simulink model "C28069_LLC_ePWM_V8_230307_PhaeShiftWorking"  (R2022b)
settings: Solver=FixedStepAuto  StartTime=0.0  StopTime=10  RelTol=1e-3  EnableMultiTasking=on
model workspace (MAT data in the model file):
  Comp_DAC = 512
undefined symbols (not defined in the file or in its folder): Down, GPTRIP1SEL, GPTRIP2SEL, PWM_Control, PWM_Gen, PWM_Gen1, SCI_A_Transmit, SCI_A_Transmit_Current_Suffix, SCI_A_Transmit_Duty_Suffix, SCI_A_Transmit_Freq_Suffix, SCI_A_Transmit_OVPFlag_Suffix, SCI_A_Transmit_PFC_Suffix, SCI_A_Transmit_SS_Suffix, SCI_A_Transmit_TBPHS_Suffix, SCI_A_Transmit_VADC_Suffix, SCI_A_Transmit_VAvg_Suffix, SCI_A_Transmit_VBAT_Suffix, SCI_A_Transmit_VBATRef_Suffix, SCI_A_Transmit_Vo_Suffix, TZ1, TZ2, u1, Up
libraries: c2802xlib x92, c280xlib x39, simulink x36, c2000lib x1
(part 2 of 18)

== system C28069_LLC_ePWM_V8_230307_PhaeShiftWorking/Simulink Function1 ==
  note: Added Trigger
  note: Fixing deadtime to 250ns
  note: Control CMPA/B to Zero
      | When the input is <1KHz
      | (To switch off ePWM)
  note: Frequency Input Selection
  note: Original
  PWM_Gen : TriggerPort  TriggerType=function-call  IsSimulinkFunction=on  FunctionName=PWM_Gen  FunctionVisibility=scoped  VariantControl=(inherit)
  CMPA : Display
  CMPA1 : Display
  CMPB : Display
  CMPB1 : Display
  Constant : Constant  Value=100
  Constant1 : Constant
  Constant2 : Constant
  Constant4 : Constant
  Dead time (%) : Display
  Dead time (sec) : Constant  Value=250E-9
  Divide : Product  Inputs=*/
  Gain : Gain  Gain=100
  Gain1 : Gain  Gain=1000
  Product{1..4} (4 alike) : Product
  Subsystem : Subsystem
  Subtract : Sum  Inputs=+-
  Switch : Switch  Criteria=u2 > Threshold  Threshold=1  SaturateOnIntegerOverflow=off  InputSameDT=off
  Switch1 : Switch  Criteria=u2 > Threshold  SaturateOnIntegerOverflow=off  InputSameDT=off
  TBPRD : Display
  ePWM1 : c2802xlib/ePWM  PwmType=C2000  useModule=ePWM6  ePWMxLINKTBPRD=Not Linked  periodUnits=Clock cycles  timerSource=Input port  timerPeriod_clk=294  timerPeriod_sec=0.0001  tbshadow=Counter equals to zero  countingMode=Up-Down  phaseActiveEnable=Disable  phaseDirection=Count down after sync  phaseActive=0  synchronizationEnable=off  dcaevt1Sync=off  dcbevt1Sync=off  synchronizationOption=Disable  dcbevt1SyncOut=off  dcaevt1SyncOut=off  cmpdSyncOut=off  cmpcSyncOut=off  cmpbSyncOut=off  zeroSyncOut=off  swfSyncOut=off  perSynchronizationOption=Counter equals to period (CTR=PRD)  clockPrescale=1  HSclockPrescale=1  enswap=off  ePWMxAStatus=on  ePWMxAactionLogic1=Do nothing  ePWMxAactionLogic2=Do nothing  ePWMxAactionLogic3=Set  ePWMxAactionLogic4=Do nothing  ePWMxAactionLogic5=Clear  ePWMxAactionLogic6=Do nothing  ePWMxACSFenable=off  ePWMxACSFvalue=Forcing disable  ePWMxASFreload=Zero  ePWMxBStatus=on  ePWMxBactionLogic1=Do nothing  ePWMxBactionLogic2=Do nothing  ePWMxBactionLogic3=Do nothing  ePWMxBactionLogic4=Clear  ePWMxBactionLogic5=Do nothing  ePWMxBactionLogic6=Set  ePWMxBCSFenable=off  ePWMxBCSFvalue=Forcing disable  ePWMxBSFreload=Zero  ePWNxBOutWay=off  ePWMxLINKCMPA=Not Linked  CMPAUnits=Clock cycles  CMPASource=Input port  CMPAValue_per=50  CMPAValue_clk=12  enCMPAshadow=Counter equals to zero (CTR=Zero)  ePWMxLINKCMPB=Not Linked  CMPBUnits=Clock cycles  CMPBSource=Input port  CMPBValue_per=50  CMPBValue_clk=283  enCMPBshadow=Counter equals to zero (CTR=Zero)  ePWMxLINKCMPC=Not Linked  CMPCUnits=Clock cycles  CMPCSource=Specify via dialog  CMPCValue_per=50  CMPCValue_clk=32000  enCMPCshadow=Counter equals to zero (CTR=Zero)  ePWMxLINKCMPD=Not Linked  CMPDUnits=Clock cycles  CMPDSource=Specify via dialog  CMPDValue_per=50  CMPDValue_clk=32000  enCMPDshadow=Counter equals to zero (CTR=Zero)  enableDBePWMxA=off  enableDBePWMxB=off  enhalfcycle=off  DBpolarity=Active high complementary (AHC)  DBedgeDelay=Positive  DBSource_ePWMxA=ePWMxA  DBSource_ePWMxB=ePWMxA  DBPeriodUnits=Clock cycles  DBperiodSource=Input port  REDperiod=10  FEDperiod=10  REDperiod_sec=0  FEDperiod_sec=0  LoadModeDBRED=Immediate without using shadow  LoadModeDBFED=Immediate without using shadow  adcstartModuleA=off  adcrequestEventA=First event  adcstartEventA=Counter equals to zero (CTR=Zero)  adcstartEventA_type2=Digital Compare Module A Event 1 start of conversion (DCAEVT1.soc)  adcstartModuleB=off  adcrequestEventB=First event  adcstartEventB=Counter equals to zero (CTR=Zero)  adcstartEventB_type2=Counter equals to zero (CTR=Zero)  intEn=off  intPrd=First event  intSel=Counter equals to zero (CTR=Zero)  intSel_type2=Counter equals to zero (CTR=Zero)  hrpe=off  enHRPWM=off  HRPWM_LoadMode=Counter equals to period (CTR=PRD)  HRPWM_CTLMode=Duty or Period control mode  HRPWM_EDGMode=Both edge  hrpeb=off  enHRPWMB=off  HRPWM_LoadModeB=Counter equals to zero (CTR=ZERO)  HRPWM_CTLModeB=Duty or Period control mode  HRPWM_EDGModeB=Both edge  enHRDBRED=off  enHRDBFED=off  enSFO=on  enautoconv=on  chopperEnable=off  chopperFrequency=1  chopperFirstwidth=1  chopperDuty=12.5%  tripZonesource=Specify via dialog  tzselOSHT1=off  tzselOSHT2=off  tzselOSHT3=off  tzselOSHDCAEV1=off  tzselOSHDCBEV1=off  tzselCBC1=off  tzselCBC2=off  tzselCBC3=off  tzselCBCDCAEV2=off  tzselCBCDCBEV2=off  tzselOSHT4=off  tzselOSHT5=off  tzselOSHT6=off  tzselCBC4=off  tzselCBC5=off  tzselCBC6=off  enTzOstIntr=off  enTzCbcIntr=off  enTzDCAEVT1Intr=off  enTzDCAEVT2Intr=off  enTzDCBEVT1Intr=off  enTzDCBEVT2Intr=off  ePWMxAforced=No action  ePWMxBforced=No action  DCAEVT1forced=Low  DCBEVT1forced=Low  DCAEVT2forced=No action  DCBEVT2forced=No action  dcah=COMP1OUT input  dcal=Trip Zone 1 input (TZ1)  dcbh=COMP1OUT input  dcbl=Trip Zone 1 input (TZ1)  dcah_type2=GPTRIP1SEL/(TZ1)  dcal_type2=GPTRIP2SEL/(TZ2)  dcbh_type2=GPTRIP1SEL/(TZ1)  dcbl_type2=GPTRIP2SEL/(TZ2)  gendcaevt1=DCAH=high and DCAL=don't care  gendcaevt2=Event disabled  gendcbevt1=DCBH=high and DCBL=don't care  gendcbevt2=Event disabled  dcaevt1src=DCAEVT1 with sync  dcaevt2src=DCAEVT2 with sync  dcbevt1src=DCBEVT1 with sync  dcbevt2src=DCBEVT2 with sync  pulsesel=Counter equals to zero (CTR=Zero)  blankinv=off  blankoffset=0  blankwidth=0  evsrcsel=Filtered version of DCAEVT1 (DCAEVT1FILT)  encape=off
      settings: LibrarySourceBlock=c2806xlib/ePWM
  ePWM4 : c2802xlib/ePWM  PwmType=C2000  useModule=ePWM5  ePWMxLINKTBPRD=Not Linked  periodUnits=Clock cycles  timerSource=Input port  timerPeriod_clk=294  timerPeriod_sec=0.0001  tbshadow=Counter equals to zero  countingMode=Up-Down  phaseActiveEnable=Disable  phaseDirection=Count down after sync  phaseActive=0  synchronizationEnable=off  dcaevt1Sync=off  dcbevt1Sync=off  synchronizationOption=Disable  dcbevt1SyncOut=off  dcaevt1SyncOut=off  cmpdSyncOut=off  cmpcSyncOut=off  cmpbSyncOut=off  zeroSyncOut=off  swfSyncOut=off  perSynchronizationOption=Counter equals to period (CTR=PRD)  clockPrescale=1  HSclockPrescale=1  enswap=off  ePWMxAStatus=on  ePWMxAactionLogic1=Do nothing  ePWMxAactionLogic2=Do nothing  ePWMxAactionLogic3=Set  ePWMxAactionLogic4=Do nothing  ePWMxAactionLogic5=Clear  ePWMxAactionLogic6=Do nothing  ePWMxACSFenable=off  ePWMxACSFvalue=Forcing disable  ePWMxASFreload=Zero  ePWMxBStatus=on  ePWMxBactionLogic1=Do nothing  ePWMxBactionLogic2=Do nothing  ePWMxBactionLogic3=Do nothing  ePWMxBactionLogic4=Clear  ePWMxBactionLogic5=Do nothing  ePWMxBactionLogic6=Set  ePWMxBCSFenable=off  ePWMxBCSFvalue=Forcing disable  ePWMxBSFreload=Zero  ePWNxBOutWay=off  ePWMxLINKCMPA=Not Linked  CMPAUnits=Clock cycles  CMPASource=Input port  CMPAValue_per=50  CMPAValue_clk=12  enCMPAshadow=Counter equals to zero (CTR=Zero)  ePWMxLINKCMPB=Not Linked  CMPBUnits=Clock cycles  CMPBSource=Input port  CMPBValue_per=50  CMPBValue_clk=283  enCMPBshadow=Counter equals to zero (CTR=Zero)  ePWMxLINKCMPC=Not Linked  CMPCUnits=Clock cycles  CMPCSource=Specify via dialog  CMPCValue_per=50  CMPCValue_clk=32000  enCMPCshadow=Counter equals to zero (CTR=Zero)  ePWMxLINKCMPD=Not Linked  CMPDUnits=Clock cycles  CMPDSource=Specify via dialog  CMPDValue_per=50  CMPDValue_clk=32000  enCMPDshadow=Counter equals to zero (CTR=Zero)  enableDBePWMxA=off  enableDBePWMxB=off  enhalfcycle=off  DBpolarity=Active high complementary (AHC)  DBedgeDelay=Positive  DBSource_ePWMxA=ePWMxA  DBSource_ePWMxB=ePWMxA  DBPeriodUnits=Clock cycles  DBperiodSource=Input port  REDperiod=10  FEDperiod=10  REDperiod_sec=0  FEDperiod_sec=0  LoadModeDBRED=Immediate without using shadow  LoadModeDBFED=Immediate without using shadow  adcstartModuleA=on  adcrequestEventA=First event  adcstartEventA=Counter equals to zero (CTR=Zero)  adcstartEventA_type2=Digital Compare Module A Event 1 start of conversion (DCAEVT1.soc)  adcstartModuleB=off  adcrequestEventB=First event  adcstartEventB=Counter equals to zero (CTR=Zero)  adcstartEventB_type2=Counter equals to zero (CTR=Zero)  intEn=on  intPrd=First event  intSel=Counter equals to zero (CTR=Zero)  intSel_type2=Counter equals to zero (CTR=Zero)  hrpe=off  enHRPWM=off  HRPWM_LoadMode=Counter equals to period (CTR=PRD)  HRPWM_CTLMode=Duty or Period control mode  HRPWM_EDGMode=Both edge  hrpeb=off  enHRPWMB=off  HRPWM_LoadModeB=Counter equals to zero (CTR=ZERO)  HRPWM_CTLModeB=Duty or Period control mode  HRPWM_EDGModeB=Both edge  enHRDBRED=off  enHRDBFED=off  enSFO=on  enautoconv=on  chopperEnable=off  chopperFrequency=1  chopperFirstwidth=1  chopperDuty=12.5%  tripZonesource=Specify via dialog  tzselOSHT1=off  tzselOSHT2=off  tzselOSHT3=off  tzselOSHDCAEV1=off  tzselOSHDCBEV1=off  tzselCBC1=off  tzselCBC2=off  tzselCBC3=off  tzselCBCDCAEV2=off  tzselCBCDCBEV2=off  tzselOSHT4=off  tzselOSHT5=off  tzselOSHT6=off  tzselCBC4=off  tzselCBC5=off  tzselCBC6=off  enTzOstIntr=off  enTzCbcIntr=off  enTzDCAEVT1Intr=off  enTzDCAEVT2Intr=off  enTzDCBEVT1Intr=off  enTzDCBEVT2Intr=off  ePWMxAforced=No action  ePWMxBforced=No action  DCAEVT1forced=Low  DCBEVT1forced=Low  DCAEVT2forced=No action  DCBEVT2forced=No action  dcah=COMP1OUT input  dcal=Trip Zone 1 input (TZ1)  dcbh=COMP1OUT input  dcbl=Trip Zone 1 input (TZ1)  dcah_type2=GPTRIP1SEL/(TZ1)  dcal_type2=GPTRIP2SEL/(TZ2)  dcbh_type2=GPTRIP1SEL/(TZ1)  dcbl_type2=GPTRIP2SEL/(TZ2)  gendcaevt1=DCAH=high and DCAL=don't care  gendcaevt2=Event disabled  gendcbevt1=DCBH=high and DCBL=don't care  gendcbevt2=Event disabled  dcaevt1src=DCAEVT1 with sync  dcaevt2src=DCAEVT2 with sync  dcbevt1src=DCBEVT1 with sync  dcbevt2src=DCBEVT2 with sync  pulsesel=Counter equals to zero (CTR=Zero)  blankinv=off  blankoffset=0  blankwidth=0  evsrcsel=Filtered version of DCAEVT1 (DCAEVT1FILT)  encape=off
      settings: LibrarySourceBlock=c2806xlib/ePWM
  u : ArgIn  DisableCoverage=on  OutDataTypeStr=uint16  ArgumentName=u
  wires:
  Product1/1 -> Gain/1
  Divide/1 -> Product2/2
  Product2/1 -> Subtract/2, Product3/1, CMPA/1
  Constant/1 -> Divide/2
  Subtract/1 -> Product4/1, CMPB/1
  Gain/1 -> Divide/1, Dead time (%)/1
  Subsystem/1(Out1) -> Product2/1, Subtract/1, ePWM4/1, ePWM1/1, TBPRD/1
  Gain1/1 -> Subsystem/1(In1), Product1/1
  Dead time (sec)/1 -> Product1/2
  Switch1/1 -> Switch/2, Gain1/1
  Constant1/1 -> Switch/1
  Constant2/1 -> Switch/3
  Switch/1 -> Product3/2, Product4/2
  Product3/1 -> ePWM1/2, ePWM4/2, CMPA1/1
  Product4/1 -> CMPB1/1, ePWM4/3, ePWM1/3
  u/1 -> Switch1/1, Switch1/2
  Constant4/1 -> Switch1/3

== system C28069_LLC_ePWM_V8_230307_PhaeShiftWorking/Softstart @5kHz ==
  function : TriggerPort  TriggerType=function-call  VariantControl=(inherit)
  Function-Call Generator : simulink/Ports & Subsystems/Function-Call Generator  sample_time=-1  numberOfIterations=1  DisallowWideOutput=off
  Function-Call Split : FunctionCallSplit  IconShape=distinctive  NumOutputPorts=4  OutputPortLayout=default
  "GetADC, FaultProtection, SoftStart  @5KHz" : Subsystem  TreatAsAtomicUnit=on
  wires:
  Function-Call Generator/1 -> Function-Call Split/1
  Function-Call Split/1 -> "GetADC, FaultProtection, SoftStart  @5KHz"/Trigger

== system C28069_LLC_ePWM_V8_230307_PhaeShiftWorking/UART Reporting @ 1Hz ==
  note: For SCI_A
  function : TriggerPort  TriggerType=function-call  VariantControl=(inherit)
  Function-Call Generator : simulink/Ports & Subsystems/Function-Call Generator  sample_time=-1  numberOfIterations=1  DisallowWideOutput=off
  Function-Call Split : FunctionCallSplit  IconShape=distinctive  NumOutputPorts=12  OutputPortLayout=default
  SCI_A_Transmit_function1 : Subsystem  TreatAsAtomicUnit=on
  SCI_A_Transmit_function10 : Subsystem  Commented=on  TreatAsAtomicUnit=on
  SCI_A_Transmit_function11 : Subsystem  Commented=on  TreatAsAtomicUnit=on
  SCI_A_Transmit_function12 : Subsystem  Commented=on  TreatAsAtomicUnit=on
  SCI_A_Transmit_function13 : Subsystem  Commented=on  TreatAsAtomicUnit=on
  SCI_A_Transmit_function14 : Subsystem  Commented=on  TreatAsAtomicUnit=on
  SCI_A_Transmit_function15 : Subsystem  TreatAsAtomicUnit=on
  SCI_A_Transmit_function16 : Subsystem  Commented=on  TreatAsAtomicUnit=on
  SCI_A_Transmit_function17 : Subsystem  TreatAsAtomicUnit=on
  SCI_A_Transmit_function18 : Subsystem  Commented=on  TreatAsAtomicUnit=on
  SCI_A_Transmit_function19 : Subsystem  TreatAsAtomicUnit=on
  SCI_A_Transmit_function2 : Subsystem  TreatAsAtomicUnit=on
  SCI_A_Transmit_function20 : Subsystem  Commented=on  TreatAsAtomicUnit=on
  SCI_A_Transmit_function21 : Subsystem  TreatAsAtomicUnit=on
  SCI_A_Transmit_function22 : Subsystem  TreatAsAtomicUnit=on
  SCI_A_Transmit_function23 : Subsystem  TreatAsAtomicUnit=on
  SCI_A_Transmit_function3 : Subsystem  TreatAsAtomicUnit=on
  SCI_A_Transmit_function4 : Subsystem  TreatAsAtomicUnit=on
  SCI_A_Transmit_function5 : Subsystem  TreatAsAtomicUnit=on
  SCI_A_Transmit_function6 : Subsystem  TreatAsAtomicUnit=on
  SCI_A_Transmit_function7 : Subsystem  TreatAsAtomicUnit=on
  SCI_A_Transmit_function8 : Subsystem  Commented=on  TreatAsAtomicUnit=on
  SCI_A_Transmit_function9 : Subsystem  Commented=on  TreatAsAtomicUnit=on
  Send Current : Subsystem  TreatAsAtomicUnit=on
  Send Duty : Subsystem  TreatAsAtomicUnit=on
  Send Freq : Subsystem  TreatAsAtomicUnit=on
  Send OVPFlag : Subsystem  Commented=on  TreatAsAtomicUnit=on
  Send PFC_OK : Subsystem  TreatAsAtomicUnit=on
  Send SoftStart : Subsystem  TreatAsAtomicUnit=on
  Send TBPHS (PhaseShift) : Subsystem  TreatAsAtomicUnit=on
  Send VADC_Avg : Subsystem  Commented=on  TreatAsAtomicUnit=on
  Send VBAT Value (Vout) : Subsystem  TreatAsAtomicUnit=on
  Send VBAT Value (Vout)1 : Subsystem  TreatAsAtomicUnit=on
  Send Vo Value : Subsystem  Commented=on  TreatAsAtomicUnit=on
  Send Voltage ADC Value : Subsystem  Commented=on  TreatAsAtomicUnit=on
  wires:
  Function-Call Split/1 -> Send Voltage ADC Value/Trigger
  Function-Call Generator/1 -> Function-Call Split/1
  Function-Call Split/7 -> Send PFC_OK/Trigger
  Function-Call Split/6 -> Send Vo Value/Trigger
  Function-Call Split/2 -> Send VADC_Avg/Trigger
  Function-Call Split/3 -> Send VBAT Value (Vout)/Trigger
  Function-Call Split/4 -> Send Freq/Trigger
  Function-Call Split/8 -> Send Current/Trigger
  Function-Call Split/5 -> Send Duty/Trigger
  Function-Call Split/9 -> Send OVPFlag/Trigger
  Function-Call Split/10 -> Send VBAT Value (Vout)1/Trigger
  Function-Call Split/11 -> Send SoftStart/Trigger
  Function-Call Split/12 -> Send TBPHS (PhaseShift)/Trigger

== system C28069_LLC_ePWM_V8_230307_PhaeShiftWorking/CloseLoop & Update @ ADCINT, 50kHz/Close Loop Regulation1 ==
  function : TriggerPort  TriggerType=function-call  VariantControl=(inherit)
  Constant : Constant
  Data Store Read1 : DataStoreRead  DataStoreName=SoftStart_OK_Signal  IndexOptions=Index vector (dialog)  Indices=1  OutputSizes=1
  Data Store Read4 : DataStoreRead  DataStoreName=PFC_OK  IndexOptions=Index vector (dialog)  Indices=1  OutputSizes=1
  If : If  NumInputs=2  IfExpression=(u1 == 1) & (u2 == 1)  ShowElse=off
  If Action Subsystem : Subsystem  TreatAsAtomicUnit=on
  wires:
  Constant/1 -> If/2
  If/1 -> If Action Subsystem/Action
  Data Store Read4/1 -> If/1

== system C28069_LLC_ePWM_V8_230307_PhaeShiftWorking/CloseLoop & Update @ ADCINT, 50kHz/Close Loop Regulation2 ==
  function : TriggerPort  TriggerType=function-call  VariantControl=(inherit)
  Data Store Read4 : DataStoreRead  DataStoreName=PFC_OK  IndexOptions=Index vector (dialog)  Indices=1  OutputSizes=1
  If : If  IfExpression=(u1 == 1)  ShowElse=off
  If Action Subsystem : Subsystem  TreatAsAtomicUnit=on
  wires:
  Data Store Read4/1 -> If/1
  If/1 -> If Action Subsystem/Action

== system C28069_LLC_ePWM_V8_230307_PhaeShiftWorking/CloseLoop & Update @ ADCINT, 50kHz/Control ==
  Action Port : ActionPort  ActionPortLabel=case [ 10 ]:
  Close Loop Regulation : Subsystem  TreatAsAtomicUnit=on
  Debug : Subsystem  Commented=on  TreatAsAtomicUnit=on
  Debug1 : Subsystem  Commented=on  TreatAsAtomicUnit=on
  Frequency Update : Subsystem  TreatAsAtomicUnit=on
  Function-Call Generator : simulink/Ports & Subsystems/Function-Call Generator  sample_time=-1  numberOfIterations=1  DisallowWideOutput=off
  Function-Call Split : FunctionCallSplit  IconShape=distinctive  NumOutputPorts=5  OutputPortLayout=default
  Get AVG2 : Subsystem  Commented=on  TreatAsAtomicUnit=on
  wires:
  Function-Call Split/3 -> Close Loop Regulation/Trigger
  Function-Call Split/4 -> Frequency Update/Trigger
  Function-Call Generator/1 -> Function-Call Split/1
  Function-Call Split/1 -> Debug/Trigger
  Function-Call Split/2 -> Get AVG2/Trigger
  Function-Call Split/5 -> Debug1/Trigger

== system C28069_LLC_ePWM_V8_230307_PhaeShiftWorking/CloseLoop & Update @ ADCINT, 50kHz/Debug2 ==
  function : TriggerPort  TriggerType=function-call  VariantControl=(inherit)
  Constant3 : Constant
  GPIO21 : c280xlib/Digital Output  GPIO_Number=GPIO16~GPIO23  GPIO_Bit0=off  GPIO_BIT0_Toggle=off  GPIO_Bit1=off  GPIO_BIT1_Toggle=off  GPIO_Bit2=off  GPIO_BIT2_Toggle=off  GPIO_Bit3=off  GPIO_BIT3_Toggle=off  GPIO_Bit4=off  GPIO_BIT4_Toggle=off  GPIO_Bit5=on  GPIO_BIT5_Toggle=off  GPIO_Bit6=off  GPIO_BIT6_Toggle=off  GPIO_Bit7=off  GPIO_BIT7_Toggle=off
  wires:
  Constant3/1 -> GPIO21/1

== system C28069_LLC_ePWM_V8_230307_PhaeShiftWorking/CloseLoop & Update @ ADCINT, 50kHz/Debug3 ==
  function : TriggerPort  TriggerType=function-call  VariantControl=(inherit)
  Constant3 : Constant  Value=0
  GPIO21 : c280xlib/Digital Output  GPIO_Number=GPIO16~GPIO23  GPIO_Bit0=off  GPIO_BIT0_Toggle=off  GPIO_Bit1=off  GPIO_BIT1_Toggle=off  GPIO_Bit2=off  GPIO_BIT2_Toggle=off  GPIO_Bit3=off  GPIO_BIT3_Toggle=off  GPIO_Bit4=off  GPIO_BIT4_Toggle=off  GPIO_Bit5=on  GPIO_BIT5_Toggle=off  GPIO_Bit6=off  GPIO_BIT6_Toggle=off  GPIO_Bit7=off  GPIO_BIT7_Toggle=off
  wires:
  Constant3/1 -> GPIO21/1

== system C28069_LLC_ePWM_V8_230307_PhaeShiftWorking/CloseLoop & Update @ ADCINT, 50kHz/Frequency Update ==
  note: Final Block for Regulation can control (sweep) frequency & dutycycle
  function : TriggerPort  TriggerType=function-call  VariantControl=(inherit)
  Constant1 : Constant  OutDataTypeStr=double
  Constant2 : Constant  Value=0  OutDataTypeStr=double
  Constant3 : Constant  Commented=on  Value=0  OutDataTypeStr=double
  Data Store Read : DataStoreRead  DataStoreName=TBPHS  IndexOptions=Index vector (dialog)  Indices=1  OutputSizes=1
  Data Store Read11 : DataStoreRead  DataStoreName=Freq_Value  IndexOptions=Index vector (dialog)  Indices=1  OutputSizes=1
  Data Store Read12 : DataStoreRead  DataStoreName=PFC_OK  IndexOptions=Index vector (dialog)  Indices=1  OutputSizes=1
  Data Store Read13 : DataStoreRead  Commented=on  DataStoreName=OVP_Flag  IndexOptions=Index vector (dialog)  Indices=1  OutputSizes=1
  Data Store Read14 : DataStoreRead  DataStoreName=Freq_Value_Out  IndexOptions=Index vector (dialog)  Indices=1  OutputSizes=1
  Data Store Read15 : DataStoreRead  Commented=on  DataStoreName=OCP_Flag  IndexOptions=Index vector (dialog)  Indices=1  OutputSizes=1
  Data Store Read16 : DataStoreRead  Commented=on  DataStoreName=Duty_Value  IndexOptions=Index vector (dialog)  Indices=1  OutputSizes=1
  Data Store Write2 : DataStoreWrite  DataStoreName=Freq_Value_Out  IndexOptions=Index vector (dialog)  Indices=1  OutputSizes=1
  Function Caller2 : FunctionCaller  FunctionPrototype=PWM_Control(u,u1)  InputArgumentSpecifications=<Enter example>  OutputArgumentSpecifications=<Enter example>
  Product2 : Product  Inputs=4  OutDataTypeStr=double
  Simulink Function1 : Subsystem  Commented=on  TreatAsAtomicUnit=on
  Simulink Function2 : Subsystem  Commented=on  TreatAsAtomicUnit=on
  Simulink Function3 : Subsystem  TreatAsAtomicUnit=on
  Switch2 : Switch  Criteria=u2 > Threshold  OutDataTypeStr=double  SaturateOnIntegerOverflow=off  InputSameDT=off
  wires:
  Switch2/1 -> Data Store Write2/1
  Data Store Read14/1 -> Function Caller2/1
  Constant2/1 -> Switch2/3
  Data Store Read12/1 -> Product2/2
  Product2/1 -> Switch2/2, Switch2/1
  Data Store Read11/1 -> Product2/1
  Constant1/1 -> Product2/4, Product2/3
  Data Store Read/1 -> Function Caller2/2

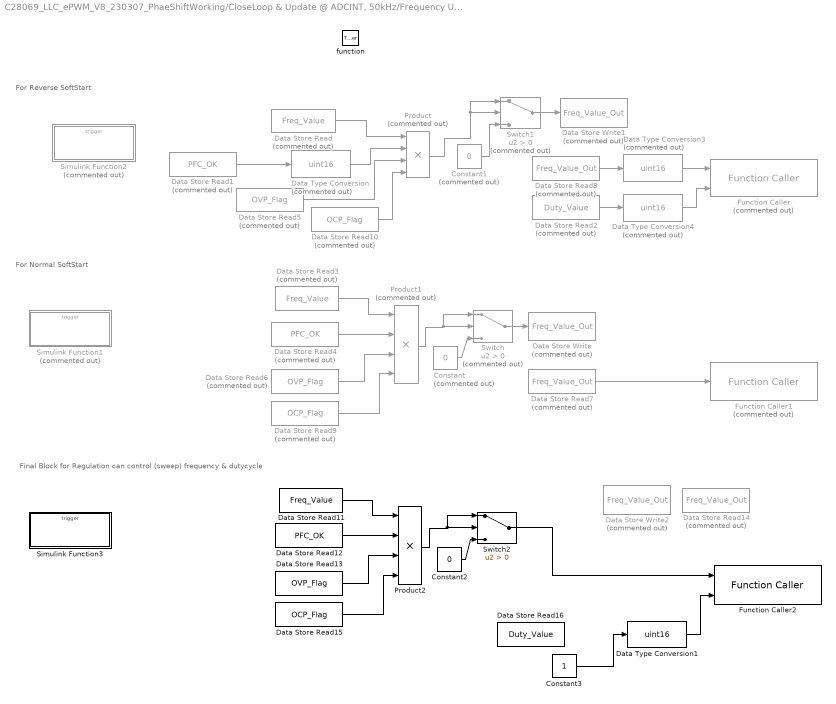
== system C28069_LLC_ePWM_V8_230307_PhaeShiftWorking/CloseLoop & Update @ ADCINT, 50kHz/Frequency Update1 ==
  note: For Reverse SoftStart
  note: For Normal SoftStart
  note: Final Block for Regulation can control (sweep) frequency & dutycycle
  function : TriggerPort  TriggerType=function-call  VariantControl=(inherit)
  Constant : Constant  Commented=on  Value=0  OutDataTypeStr=double
  Constant1 : Constant  Commented=on  Value=0
  Constant2 : Constant  Value=0  OutDataTypeStr=double
  Constant3 : Constant  OutDataTypeStr=double
  Data Store Read : DataStoreRead  Commented=on  DataStoreName=Freq_Value  IndexOptions=Index vector (dialog)  Indices=1  OutputSizes=1
  Data Store Read1 : DataStoreRead  Commented=on  DataStoreName=PFC_OK  IndexOptions=Index vector (dialog)  Indices=1  OutputSizes=1
  Data Store Read10 : DataStoreRead  Commented=on  DataStoreName=OCP_Flag  IndexOptions=Index vector (dialog)  Indices=1  OutputSizes=1
  Data Store Read11 : DataStoreRead  DataStoreName=Freq_Value  IndexOptions=Index vector (dialog)  Indices=1  OutputSizes=1
  Data Store Read12 : DataStoreRead  DataStoreName=PFC_OK  IndexOptions=Index vector (dialog)  Indices=1  OutputSizes=1
  Data Store Read13 : DataStoreRead  DataStoreName=OVP_Flag  IndexOptions=Index vector (dialog)  Indices=1  OutputSizes=1
  Data Store Read14 : DataStoreRead  Commented=on  DataStoreName=Freq_Value_Out  IndexOptions=Index vector (dialog)  Indices=1  OutputSizes=1
  Data Store Read15 : DataStoreRead  DataStoreName=OCP_Flag  IndexOptions=Index vector (dialog)  Indices=1  OutputSizes=1
  Data Store Read16 : DataStoreRead  DataStoreName=Duty_Value  IndexOptions=Index vector (dialog)  Indices=1  OutputSizes=1
  Data Store Read2 : DataStoreRead  Commented=on  DataStoreName=Duty_Value  IndexOptions=Index vector (dialog)  Indices=1  OutputSizes=1
  Data Store Read3 : DataStoreRead  Commented=on  DataStoreName=Freq_Value  IndexOptions=Index vector (dialog)  Indices=1  OutputSizes=1
  Data Store Read4 : DataStoreRead  Commented=on  DataStoreName=PFC_OK  IndexOptions=Index vector (dialog)  Indices=1  OutputSizes=1
  Data Store Read5 : DataStoreRead  Commented=on  DataStoreName=OVP_Flag  IndexOptions=Index vector (dialog)  Indices=1  OutputSizes=1
  Data Store Read6 : DataStoreRead  Commented=on  DataStoreName=OVP_Flag  IndexOptions=Index vector (dialog)  Indices=1  OutputSizes=1
  Data Store Read7 : DataStoreRead  Commented=on  DataStoreName=Freq_Value_Out  IndexOptions=Index vector (dialog)  Indices=1  OutputSizes=1
  Data Store Read8 : DataStoreRead  Commented=on  DataStoreName=Freq_Value_Out  IndexOptions=Index vector (dialog)  Indices=1  OutputSizes=1
  Data Store Read9 : DataStoreRead  Commented=on  DataStoreName=OCP_Flag  IndexOptions=Index vector (dialog)  Indices=1  OutputSizes=1
  Data Store Write : DataStoreWrite  Commented=on  DataStoreName=Freq_Value_Out  IndexOptions=Index vector (dialog)  Indices=1  OutputSizes=1
  Data Store Write1 : DataStoreWrite  Commented=on  DataStoreName=Freq_Value_Out  IndexOptions=Index vector (dialog)  Indices=1  OutputSizes=1
  Data Store Write2 : DataStoreWrite  Commented=on  DataStoreName=Freq_Value_Out  IndexOptions=Index vector (dialog)  Indices=1  OutputSizes=1
  Data Type Conversion : DataTypeConversion  Commented=on  OutDataTypeStr=uint16  SaturateOnIntegerOverflow=off  RndMeth=Floor
  Data Type Conversion1 : DataTypeConversion  OutDataTypeStr=uint16  SaturateOnIntegerOverflow=off  RndMeth=Floor
  Data Type Conversion3 : DataTypeConversion  Commented=on  OutDataTypeStr=uint16  SaturateOnIntegerOverflow=off  RndMeth=Floor
  Data Type Conversion4 : DataTypeConversion  Commented=on  OutDataTypeStr=uint16  SaturateOnIntegerOverflow=off  RndMeth=Floor
  Function Caller : FunctionCaller  Commented=on  FunctionPrototype=PWM_Gen1(u,u1)  InputArgumentSpecifications=<Enter example>  OutputArgumentSpecifications=<Enter example>
  Function Caller1 : FunctionCaller  Commented=on  FunctionPrototype=PWM_Gen(u)  InputArgumentSpecifications=<Enter example>  OutputArgumentSpecifications=<Enter example>
  Function Caller2 : FunctionCaller  FunctionPrototype=PWM_Control(u,u1)  InputArgumentSpecifications=<Enter example>  OutputArgumentSpecifications=<Enter example>
  Product : Product  Commented=on  Inputs=4  OutDataTypeStr=uint16
  Product1 : Product  Commented=on  Inputs=4  OutDataTypeStr=double
  Product2 : Product  Inputs=4  OutDataTypeStr=double
  Simulink Function1 : Subsystem  Commented=on  TreatAsAtomicUnit=on
  Simulink Function2 : Subsystem  Commented=on  TreatAsAtomicUnit=on
  Simulink Function3 : Subsystem  TreatAsAtomicUnit=on
  Switch : Switch  Commented=on  Criteria=u2 > Threshold  OutDataTypeStr=double  SaturateOnIntegerOverflow=off  InputSameDT=off
  Switch1 : Switch  Commented=on  Criteria=u2 > Threshold  SaturateOnIntegerOverflow=off  InputSameDT=off
  Switch2 : Switch  Criteria=u2 > Threshold  OutDataTypeStr=double  SaturateOnIntegerOverflow=off  InputSameDT=off
  wires:
  Data Store Read1/1 -> Data Type Conversion/1
  Data Type Conversion/1 -> Product/2
  Data Store Read7/1 -> Function Caller1/1
  Product1/1 -> Switch/2, Switch/1
  Data Store Read2/1 -> Data Type Conversion4/1
  Data Store Read10/1 -> Product/4
  Data Store Read5/1 -> Product/3
  Constant1/1 -> Switch1/3
  Data Store Read4/1 -> Product1/2
  Data Store Read/1 -> Product/1
  Product/1 -> Switch1/2, Switch1/1
  Data Store Read9/1 -> Product1/4
  Constant/1 -> Switch/3
  Data Type Conversion3/1 -> Function Caller/1
  Data Store Read6/1 -> Product1/3
  Switch1/1 -> Data Store Write1/1
  Switch/1 -> Data Store Write/1
  Data Type Conversion4/1 -> Function Caller/2
  Data Store Read3/1 -> Product1/1
  Data Store Read8/1 -> Data Type Conversion3/1
  Constant2/1 -> Switch2/3
  Data Store Read11/1 -> Product2/1
  Data Store Read15/1 -> Product2/4
  Data Store Read13/1 -> Product2/3
  Product2/1 -> Switch2/2, Switch2/1
  Data Store Read12/1 -> Product2/2
  Data Type Conversion1/1 -> Function Caller2/2
  Constant3/1 -> Data Type Conversion1/1
  Switch2/1 -> Function Caller2/1

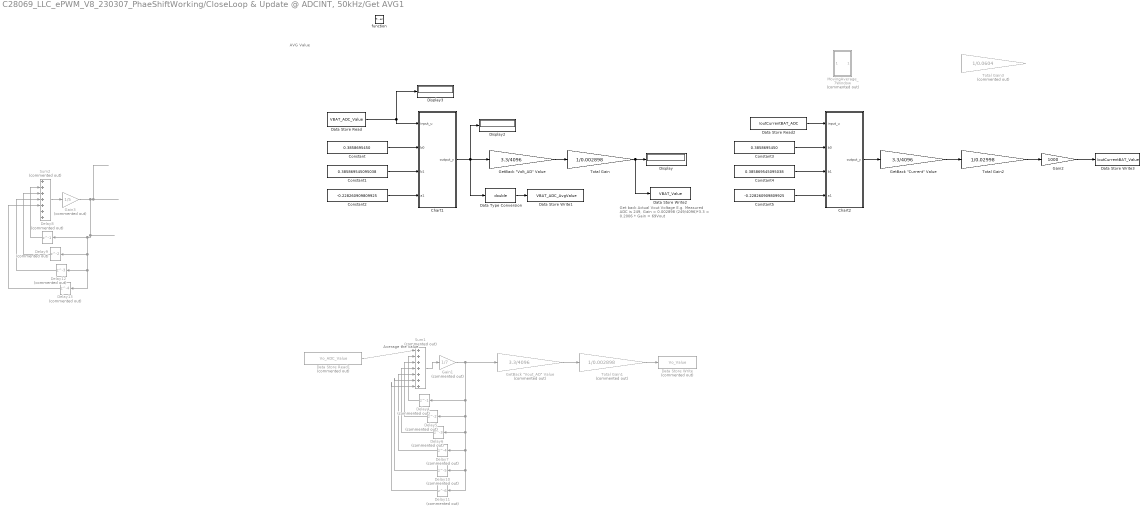
== system C28069_LLC_ePWM_V8_230307_PhaeShiftWorking/CloseLoop & Update @ ADCINT, 50kHz/Get AVG1 ==
  note: AVG Value
  note: Average the value
  note: Get back Actual Vout Voltage
      | E.g.
      | Measured ADC is 249, Gain = 0.002898
      | (249/4096)*3.3 = 0.2006 * Gain
      | = 69Vout
  function : TriggerPort  TriggerType=function-call  VariantControl=(inherit)
  Chart1 : Stateflow chart  TreatAsAtomicUnit=on
  Chart2 : Stateflow chart  TreatAsAtomicUnit=on
  Constant : Constant  Value=0.3858695450
  Constant1 : Constant  Value=0.385869545095038
  Constant2 : Constant  Value=-0.228260909809925
  Constant3 : Constant  Value=0.3858695450
  Constant4 : Constant  Value=0.385869545095038
  Constant5 : Constant  Value=-0.228260909809925
  Data Store Read : DataStoreRead  DataStoreName=VBAT_ADC_Value  IndexOptions=Index vector (dialog)  Indices=1  OutputSizes=1
  Data Store Read1 : DataStoreRead  Commented=on  DataStoreName=Vo_ADC_Value  IndexOptions=Index vector (dialog)  Indices=1  OutputSizes=1
  Data Store Read2 : DataStoreRead  DataStoreName=IoutCurrentBAT_ADC  IndexOptions=Index vector (dialog)  Indices=1  OutputSizes=1
  Data Store Write : DataStoreWrite  Commented=on  DataStoreName=Vo_Value  IndexOptions=Index vector (dialog)  Indices=1  OutputSizes=1
  Data Store Write1 : DataStoreWrite  DataStoreName=VBAT_ADC_AvgValue  IndexOptions=Index vector (dialog)  Indices=1  OutputSizes=1
  Data Store Write2 : DataStoreWrite  DataStoreName=VBAT_Value  IndexOptions=Index vector (dialog)  Indices=1  OutputSizes=1
  Data Store Write3 : DataStoreWrite  DataStoreName=IoutCurrentBAT_Value  IndexOptions=Index vector (dialog)  Indices=1  OutputSizes=1
  Data Type Conversion : DataTypeConversion  OutDataTypeStr=double  SaturateOnIntegerOverflow=off  RndMeth=Floor
  Delay10 : Delay  Commented=on  DelayLength=5
  Delay11 : Delay  Commented=on  DelayLength=6
  Delay12 : Delay  Commented=on  DelayLength=3
  Delay13 : Delay  Commented=on  DelayLength=4
  Delay4 : Delay  Commented=on  DelayLength=1
  Delay5 : Delay  Commented=on
  Delay6 : Delay  Commented=on  DelayLength=3
  Delay7 : Delay  Commented=on  DelayLength=4
  Delay8 : Delay  Commented=on  DelayLength=1
  Delay9 : Delay  Commented=on
  Display : Display
      settings: Decimation=2
  Display2 : Display
  Display3 : Display
  Gain1 : Gain  Commented=on  Gain=1/7  OutDataTypeStr=uint16
  Gain2 : Gain  Gain=1000
  Gain3 : Gain  Commented=on  Gain=1/5  OutDataTypeStr=uint16
  "GetBack \"Current\" Value" : Gain  Gain=3.3/4096  OutDataTypeStr=double
  "GetBack \"Volt_AD\" Value" : Gain  Gain=3.3/4096  OutDataTypeStr=double
  "GetBack \"Vout_AD\" Value" : Gain  Commented=on  Gain=3.3/4096  OutDataTypeStr=double
  MovingAverage_7Window : Subsystem  Commented=on
  Sum1 : Sum  Commented=on  Inputs=|+++++++
  Sum2 : Sum  Commented=on  Inputs=|+++++++
  Total Gain : Gain  Gain=1/0.002898  OutDataTypeStr=double
  Total Gain1 : Gain  Commented=on  Gain=1/0.002898  OutDataTypeStr=double
  Total Gain2 : Gain  Gain=1/0.02998  OutDataTypeStr=double
  Total Gain3 : Gain  Commented=on  Gain=1/0.0604  OutDataTypeStr=double
  wires:
  Delay4/1 -> Sum1/2
  Total Gain1/1 -> Data Store Write/1
  "GetBack \"Current\" Value"/1 -> Total Gain2/1
  Delay7/1 -> Sum1/5
  Gain1/1 -> Delay4/1, Delay5/1, Delay6/1, Delay7/1, Delay10/1, Delay11/1, "GetBack \"Vout_AD\" Value"/1
  Data Type Conversion/1 -> Data Store Write1/1
  Delay6/1 -> Sum1/4
  Delay11/1 -> Sum1/7
  Delay10/1 -> Sum1/6
  "GetBack \"Vout_AD\" Value"/1 -> Total Gain1/1
  "GetBack \"Volt_AD\" Value"/1 -> Total Gain/1
  Data Store Read1/1 -> Sum1/1
  Total Gain/1 -> Display/1, Data Store Write2/1
  Sum1/1 -> Gain1/1
  Delay5/1 -> Sum1/3
  Total Gain2/1 -> Gain2/1
  Gain2/1 -> Data Store Write3/1
  Gain3/1 -> Delay9/1, Delay12/1, Delay13/1, Delay8/1
  Delay9/1 -> Sum2/3
  Sum2/1 -> Gain3/1
  Delay13/1 -> Sum2/5
  Delay12/1 -> Sum2/4
  Delay8/1 -> Sum2/2
  Data Store Read/1 -> Chart1/1(input_u), Display3/1
  Constant2/1 -> Chart1/4(a1)
  Constant1/1 -> Chart1/3(b1)
  Constant/1 -> Chart1/2(b0)
  Chart1/1(output_y) -> Display2/1, Data Type Conversion/1, "GetBack \"Volt_AD\" Value"/1
  Constant3/1 -> Chart2/2(b0)
  Constant4/1 -> Chart2/3(b1)
  Constant5/1 -> Chart2/4(a1)
  Data Store Read2/1 -> Chart2/1(input_u)
  Chart2/1(output_y) -> "GetBack \"Current\" Value"/1

== system C28069_LLC_ePWM_V8_230307_PhaeShiftWorking/GetADC Measurement @50KHz3/Close Loop Regulation ==
  function : TriggerPort  TriggerType=function-call  VariantControl=(inherit)
  Constant : Constant
  Data Store Read1 : DataStoreRead  DataStoreName=SoftStart_OK_Signal  IndexOptions=Index vector (dialog)  Indices=1  OutputSizes=1
  Data Store Read4 : DataStoreRead  DataStoreName=PFC_OK  IndexOptions=Index vector (dialog)  Indices=1  OutputSizes=1
  If : If  NumInputs=2  IfExpression=(u1 == 1) & (u2 == 1)  ShowElse=off
  If Action Subsystem : Subsystem  TreatAsAtomicUnit=on
  wires:
  Data Store Read4/1 -> If/1
  If/1 -> If Action Subsystem/Action
  Constant/1 -> If/2

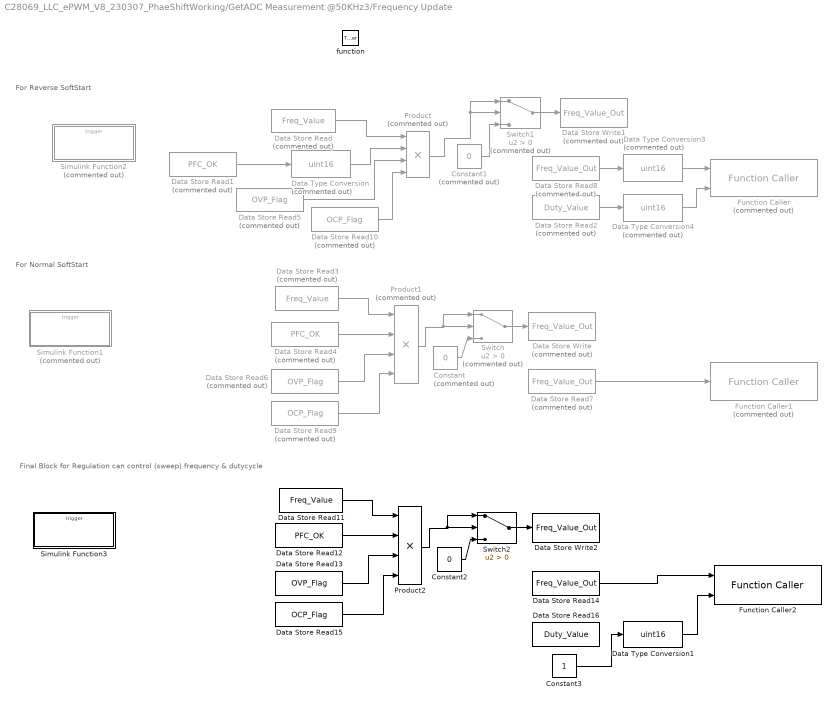
== system C28069_LLC_ePWM_V8_230307_PhaeShiftWorking/GetADC Measurement @50KHz3/Frequency Update ==
  note: Final Block for Regulation can control (sweep) frequency & dutycycle
  note: For Normal SoftStart
  note: For Reverse SoftStart
  function : TriggerPort  TriggerType=function-call  VariantControl=(inherit)
  Constant : Constant  Commented=on  Value=0  OutDataTypeStr=double
  Constant1 : Constant  Commented=on  Value=0
  Constant2 : Constant  Value=0  OutDataTypeStr=double
  Constant3 : Constant  OutDataTypeStr=double
  Data Store Read : DataStoreRead  Commented=on  DataStoreName=Freq_Value  IndexOptions=Index vector (dialog)  Indices=1  OutputSizes=1
  Data Store Read1 : DataStoreRead  Commented=on  DataStoreName=PFC_OK  IndexOptions=Index vector (dialog)  Indices=1  OutputSizes=1
  Data Store Read10 : DataStoreRead  Commented=on  DataStoreName=OCP_Flag  IndexOptions=Index vector (dialog)  Indices=1  OutputSizes=1
  Data Store Read11 : DataStoreRead  DataStoreName=Freq_Value  IndexOptions=Index vector (dialog)  Indices=1  OutputSizes=1
  Data Store Read12 : DataStoreRead  DataStoreName=PFC_OK  IndexOptions=Index vector (dialog)  Indices=1  OutputSizes=1
  Data Store Read13 : DataStoreRead  DataStoreName=OVP_Flag  IndexOptions=Index vector (dialog)  Indices=1  OutputSizes=1
  Data Store Read14 : DataStoreRead  DataStoreName=Freq_Value_Out  IndexOptions=Index vector (dialog)  Indices=1  OutputSizes=1
  Data Store Read15 : DataStoreRead  DataStoreName=OCP_Flag  IndexOptions=Index vector (dialog)  Indices=1  OutputSizes=1
  Data Store Read16 : DataStoreRead  DataStoreName=Duty_Value  IndexOptions=Index vector (dialog)  Indices=1  OutputSizes=1
  Data Store Read2 : DataStoreRead  Commented=on  DataStoreName=Duty_Value  IndexOptions=Index vector (dialog)  Indices=1  OutputSizes=1
  Data Store Read3 : DataStoreRead  Commented=on  DataStoreName=Freq_Value  IndexOptions=Index vector (dialog)  Indices=1  OutputSizes=1
  Data Store Read4 : DataStoreRead  Commented=on  DataStoreName=PFC_OK  IndexOptions=Index vector (dialog)  Indices=1  OutputSizes=1
  Data Store Read5 : DataStoreRead  Commented=on  DataStoreName=OVP_Flag  IndexOptions=Index vector (dialog)  Indices=1  OutputSizes=1
  Data Store Read6 : DataStoreRead  Commented=on  DataStoreName=OVP_Flag  IndexOptions=Index vector (dialog)  Indices=1  OutputSizes=1
  Data Store Read7 : DataStoreRead  Commented=on  DataStoreName=Freq_Value_Out  IndexOptions=Index vector (dialog)  Indices=1  OutputSizes=1
  Data Store Read8 : DataStoreRead  Commented=on  DataStoreName=Freq_Value_Out  IndexOptions=Index vector (dialog)  Indices=1  OutputSizes=1
  Data Store Read9 : DataStoreRead  Commented=on  DataStoreName=OCP_Flag  IndexOptions=Index vector (dialog)  Indices=1  OutputSizes=1
  Data Store Write : DataStoreWrite  Commented=on  DataStoreName=Freq_Value_Out  IndexOptions=Index vector (dialog)  Indices=1  OutputSizes=1
  Data Store Write1 : DataStoreWrite  Commented=on  DataStoreName=Freq_Value_Out  IndexOptions=Index vector (dialog)  Indices=1  OutputSizes=1
  Data Store Write2 : DataStoreWrite  DataStoreName=Freq_Value_Out  IndexOptions=Index vector (dialog)  Indices=1  OutputSizes=1
  Data Type Conversion : DataTypeConversion  Commented=on  OutDataTypeStr=uint16  SaturateOnIntegerOverflow=off  RndMeth=Floor
  Data Type Conversion1 : DataTypeConversion  OutDataTypeStr=uint16  SaturateOnIntegerOverflow=off  RndMeth=Floor
  Data Type Conversion3 : DataTypeConversion  Commented=on  OutDataTypeStr=uint16  SaturateOnIntegerOverflow=off  RndMeth=Floor
  Data Type Conversion4 : DataTypeConversion  Commented=on  OutDataTypeStr=uint16  SaturateOnIntegerOverflow=off  RndMeth=Floor
  Function Caller : FunctionCaller  Commented=on  FunctionPrototype=PWM_Gen1(u,u1)  InputArgumentSpecifications=<Enter example>  OutputArgumentSpecifications=<Enter example>
  Function Caller1 : FunctionCaller  Commented=on  FunctionPrototype=PWM_Gen(u)  InputArgumentSpecifications=<Enter example>  OutputArgumentSpecifications=<Enter example>
  Function Caller2 : FunctionCaller  FunctionPrototype=PWM_Control(u,u1)  InputArgumentSpecifications=<Enter example>  OutputArgumentSpecifications=<Enter example>
  Product : Product  Commented=on  Inputs=4  OutDataTypeStr=uint16
  Product1 : Product  Commented=on  Inputs=4  OutDataTypeStr=double
  Product2 : Product  Inputs=4  OutDataTypeStr=double
  Simulink Function1 : Subsystem  Commented=on  TreatAsAtomicUnit=on
  Simulink Function2 : Subsystem  Commented=on  TreatAsAtomicUnit=on
  Simulink Function3 : Subsystem  TreatAsAtomicUnit=on
  Switch : Switch  Commented=on  Criteria=u2 > Threshold  OutDataTypeStr=double  SaturateOnIntegerOverflow=off  InputSameDT=off
  Switch1 : Switch  Commented=on  Criteria=u2 > Threshold  SaturateOnIntegerOverflow=off  InputSameDT=off
  Switch2 : Switch  Criteria=u2 > Threshold  OutDataTypeStr=double  SaturateOnIntegerOverflow=off  InputSameDT=off
  wires:
  Constant3/1 -> Data Type Conversion1/1
  Data Type Conversion1/1 -> Function Caller2/2
  Data Store Read14/1 -> Function Caller2/1
  Data Store Read12/1 -> Product2/2
  Product2/1 -> Switch2/1, Switch2/2
  Data Store Read13/1 -> Product2/3
  Data Store Read15/1 -> Product2/4
  Switch2/1 -> Data Store Write2/1
  Data Store Read11/1 -> Product2/1
  Constant2/1 -> Switch2/3
  Data Store Read8/1 -> Data Type Conversion3/1
  Data Store Read3/1 -> Product1/1
  Data Type Conversion4/1 -> Function Caller/2
  Switch/1 -> Data Store Write/1
  Switch1/1 -> Data Store Write1/1
  Data Store Read6/1 -> Product1/3
  Data Type Conversion3/1 -> Function Caller/1
  Constant/1 -> Switch/3
  Data Store Read9/1 -> Product1/4
  Product/1 -> Switch1/1, Switch1/2
  Data Store Read/1 -> Product/1
  Data Store Read4/1 -> Product1/2
  Constant1/1 -> Switch1/3
  Data Store Read5/1 -> Product/3
  Data Store Read10/1 -> Product/4
  Data Store Read2/1 -> Data Type Conversion4/1
  Product1/1 -> Switch/1, Switch/2
  Data Store Read7/1 -> Function Caller1/1
  Data Type Conversion/1 -> Product/2
  Data Store Read1/1 -> Data Type Conversion/1

== system C28069_LLC_ePWM_V8_230307_PhaeShiftWorking/GetADC Measurement @50KHz3/Get ADC ==
  note: Vo ADC Measurement
  note: Current Measurement
  function : TriggerPort  TriggerType=function-call  VariantControl=(inherit)
  ADC : c2802xlib/ADC  blkParamProc=C2000  ADCModule=1  samplingMode=Single sample mode  ADCResolution=12-bit (Single-ended input)  useSOC1=SOC0  useSOC2=SOC0_SOC1  SOCAcquisitionWindow=10  SOCTriggerSource=Software  SOCInterruptTrigger=No ADCINT  Ts=-1  dType=double  postInterrupt=off  interruptSel=ADCINT1  ADCINTContinuous=off  endma=off  chdma=1  conv1=ADCINA2  conv2=ADCINA0 and ADCINB0  conv1_Type4=ADCIN0  conv2_Type4=ADCIN0 and ADCIN1
      settings: LibrarySourceBlock=c2806xlib/ADC
  ADC1 : c2802xlib/ADC  blkParamProc=C2000  ADCModule=1  samplingMode=Single sample mode  ADCResolution=12-bit (Single-ended input)  useSOC1=SOC1  useSOC2=SOC0_SOC1  SOCAcquisitionWindow=10  SOCTriggerSource=Software  SOCInterruptTrigger=No ADCINT  Ts=-1  dType=double  postInterrupt=off  interruptSel=ADCINT1  ADCINTContinuous=off  endma=off  chdma=1  conv1=ADCINA3  conv2=ADCINA0 and ADCINB0  conv1_Type4=ADCIN0  conv2_Type4=ADCIN0 and ADCIN1
      settings: LibrarySourceBlock=c2806xlib/ADC
  ADC2 : c2802xlib/ADC  blkParamProc=C2000  ADCModule=1  samplingMode=Single sample mode  ADCResolution=12-bit (Single-ended input)  useSOC1=SOC2  useSOC2=SOC0_SOC1  SOCAcquisitionWindow=10  SOCTriggerSource=Software  SOCInterruptTrigger=No ADCINT  Ts=-1  dType=double  postInterrupt=off  interruptSel=ADCINT1  ADCINTContinuous=off  endma=off  chdma=1  conv1=ADCINA0  conv2=ADCINA0 and ADCINB0  conv1_Type4=ADCIN0  conv2_Type4=ADCIN0 and ADCIN1
      settings: LibrarySourceBlock=c2806xlib/ADC
  Data Store Write : DataStoreWrite  DataStoreName=VBAT_ADC_Value  IndexOptions=Index vector (dialog)  Indices=1  OutputSizes=1
  Data Store Write1 : DataStoreWrite  DataStoreName=Vo_ADC_Value  IndexOptions=Index vector (dialog)  Indices=1  OutputSizes=1
  Data Store Write2 : DataStoreWrite  DataStoreName=IoutCurrentBAT_ADC  IndexOptions=Index vector (dialog)  Indices=1  OutputSizes=1
  wires:
  ADC/1 -> Data Store Write/1
  ADC1/1 -> Data Store Write1/1
  ADC2/1 -> Data Store Write2/1

== system C28069_LLC_ePWM_V8_230307_PhaeShiftWorking/GetADC Measurement @50KHz3/Get AVG2 ==
  note: Get back Actual Vout Voltage
      | E.g.
      | Measured ADC is 249, Gain = 0.002898
      | (249/4096)*3.3 = 0.2006 * Gain
      | = 69Vout
  note: Average the value
  note: AVG Value
  function : TriggerPort  TriggerType=function-call  VariantControl=(inherit)
  Constant : Constant  Value=249
  Data Store Read : DataStoreRead  DataStoreName=VBAT_ADC_Value  IndexOptions=Index vector (dialog)  Indices=1  OutputSizes=1
  Data Store Read1 : DataStoreRead  DataStoreName=Vo_ADC_Value  IndexOptions=Index vector (dialog)  Indices=1  OutputSizes=1
  Data Store Read2 : DataStoreRead  DataStoreName=IoutCurrentBAT_ADC  IndexOptions=Index vector (dialog)  Indices=1  OutputSizes=1
  Data Store Write : DataStoreWrite  DataStoreName=Vo_Value  IndexOptions=Index vector (dialog)  Indices=1  OutputSizes=1
  Data Store Write1 : DataStoreWrite  DataStoreName=VBAT_ADC_AvgValue  IndexOptions=Index vector (dialog)  Indices=1  OutputSizes=1
  Data Store Write2 : DataStoreWrite  DataStoreName=VBAT_Value  IndexOptions=Index vector (dialog)  Indices=1  OutputSizes=1
  Data Store Write3 : DataStoreWrite  DataStoreName=IoutCurrentBAT_Value  IndexOptions=Index vector (dialog)  Indices=1  OutputSizes=1
  Data Type Conversion : DataTypeConversion  OutDataTypeStr=double  SaturateOnIntegerOverflow=off  RndMeth=Floor
  Delay : Delay  DelayLength=1
  Delay1 : Delay
  Delay10 : Delay  DelayLength=5
  Delay11 : Delay  DelayLength=6
  Delay2 : Delay  DelayLength=3
  Delay3 : Delay  DelayLength=4
  Delay4 : Delay  DelayLength=1
  Delay5 : Delay
  Delay6 : Delay  DelayLength=3
  Delay7 : Delay  DelayLength=4
  Display : Display
      settings: Decimation=2
  Display2 : Display
  Display3 : Display
  Gain : Gain  Gain=1/5  OutDataTypeStr=uint16
  Gain1 : Gain  Gain=1/7  OutDataTypeStr=uint16
  Gain2 : Gain  Gain=1000
  "GetBack \"Current\" Value" : Gain  Gain=3.3/4096  OutDataTypeStr=double
  "GetBack \"Volt_AD\" Value" : Gain  Gain=3.3/4096  OutDataTypeStr=double
  "GetBack \"Vout_AD\" Value" : Gain  Gain=3.3/4096  OutDataTypeStr=double
  MovingAverage_7Window : Subsystem
  Sum : Sum  Inputs=|+++++++
  Sum1 : Sum  Inputs=|+++++++
  Total Gain : Gain  Gain=1/0.002898  OutDataTypeStr=double
  Total Gain1 : Gain  Gain=1/0.002898  OutDataTypeStr=double
  Total Gain2 : Gain  Gain=1/0.02998  OutDataTypeStr=double
  Total Gain3 : Gain  Commented=on  Gain=1/0.0604  OutDataTypeStr=double
  wires:
  Delay2/1 -> Sum/4
  Gain2/1 -> Data Store Write3/1
  Total Gain2/1 -> Gain2/1
  MovingAverage_7Window/1(Out1) -> "GetBack \"Current\" Value"/1
  Delay5/1 -> Sum1/3
  Sum1/1 -> Gain1/1
  Sum/1 -> Gain/1
  Delay/1 -> Sum/2
  Total Gain/1 -> Data Store Write2/1, Display/1
  Data Store Read1/1 -> Sum1/1
  "GetBack \"Volt_AD\" Value"/1 -> Total Gain/1
  "GetBack \"Vout_AD\" Value"/1 -> Total Gain1/1
  Data Store Read/1 -> Sum/1, Display3/1
  Delay10/1 -> Sum1/6
  Delay11/1 -> Sum1/7
  Delay3/1 -> Sum/5
  Data Store Read2/1 -> MovingAverage_7Window/1(In1)
  Gain/1 -> Data Type Conversion/1, "GetBack \"Volt_AD\" Value"/1, Display2/1, Delay/1, Delay3/1, Delay2/1, Delay1/1
  Delay6/1 -> Sum1/4
  Data Type Conversion/1 -> Data Store Write1/1
  Gain1/1 -> "GetBack \"Vout_AD\" Value"/1, Delay11/1, Delay10/1, Delay7/1, Delay6/1, Delay5/1, Delay4/1
  Delay7/1 -> Sum1/5
  "GetBack \"Current\" Value"/1 -> Total Gain2/1
  Total Gain1/1 -> Data Store Write/1
  Delay1/1 -> Sum/3
  Delay4/1 -> Sum1/2

== system C28069_LLC_ePWM_V8_230307_PhaeShiftWorking/GetADC Measurement @50kHz/Get ADC ==
  note: Current Measurement
  note: Vo ADC Measurement
  function : TriggerPort  TriggerType=function-call  VariantControl=(inherit)
  ADC : c2802xlib/ADC  blkParamProc=C2000  ADCModule=1  samplingMode=Single sample mode  ADCResolution=12-bit (Single-ended input)  useSOC1=SOC0  useSOC2=SOC0_SOC1  SOCAcquisitionWindow=10  SOCTriggerSource=ePWM2_ADCSOCA  SOCInterruptTrigger=No ADCINT  Ts=-1  dType=double  postInterrupt=on  interruptSel=ADCINT1  ADCINTContinuous=on  endma=off  chdma=1  conv1=ADCINA2  conv2=ADCINA0 and ADCINB0  conv1_Type4=ADCIN0  conv2_Type4=ADCIN0 and ADCIN1
      settings: LibrarySourceBlock=c2806xlib/ADC
  ADC1 : c2802xlib/ADC  Commented=on  blkParamProc=C2000  ADCModule=1  samplingMode=Single sample mode  ADCResolution=12-bit (Single-ended input)  useSOC1=SOC1  useSOC2=SOC0_SOC1  SOCAcquisitionWindow=10  SOCTriggerSource=Software  SOCInterruptTrigger=No ADCINT  Ts=-1  dType=double  postInterrupt=off  interruptSel=ADCINT1  ADCINTContinuous=off  endma=off  chdma=1  conv1=ADCINA3  conv2=ADCINA0 and ADCINB0  conv1_Type4=ADCIN0  conv2_Type4=ADCIN0 and ADCIN1
      settings: LibrarySourceBlock=c2806xlib/ADC
  ADC2 : c2802xlib/ADC  Commented=on  blkParamProc=C2000  ADCModule=1  samplingMode=Single sample mode  ADCResolution=12-bit (Single-ended input)  useSOC1=SOC2  useSOC2=SOC0_SOC1  SOCAcquisitionWindow=10  SOCTriggerSource=Software  SOCInterruptTrigger=No ADCINT  Ts=-1  dType=double  postInterrupt=on  interruptSel=ADCINT1  ADCINTContinuous=on  endma=off  chdma=1  conv1=ADCINA0  conv2=ADCINA0 and ADCINB0  conv1_Type4=ADCIN0  conv2_Type4=ADCIN0 and ADCIN1
      settings: LibrarySourceBlock=c2806xlib/ADC
  Data Store Read3 : DataStoreRead  Commented=on  DataStoreName=VBAT_ADC_Value  IndexOptions=Index vector (dialog)  Indices=1  OutputSizes=1
  Data Store Write : DataStoreWrite  Commented=on  DataStoreName=VBAT_ADC_Value  IndexOptions=Index vector (dialog)  Indices=1  OutputSizes=1
  Data Store Write1 : DataStoreWrite  Commented=on  DataStoreName=Vo_ADC_Value  IndexOptions=Index vector (dialog)  Indices=1  OutputSizes=1
  Data Store Write2 : DataStoreWrite  Commented=on  DataStoreName=IoutCurrentBAT_ADC  IndexOptions=Index vector (dialog)  Indices=1  OutputSizes=1
  Data Store Write4 : DataStoreWrite  DataStoreName=VBAT_Value  IndexOptions=Index vector (dialog)  Indices=1  OutputSizes=1
  "GetBack \"Volt_AD\" Value2" : Gain  Gain=0.278006923  OutDataTypeStr=double
  wires:
  ADC2/1 -> Data Store Write2/1
  ADC1/1 -> Data Store Write1/1
  "GetBack \"Volt_AD\" Value2"/1 -> Data Store Write4/1
  ADC/1 -> Data Store Write/1, "GetBack \"Volt_AD\" Value2"/1
